simulink model "Task2_state_feedback_controller"  (R2023b)
settings: Solver=VariableStepAuto  StartTime=0.0  StopTime=0.02  RelTol=1e-3
values from neighbouring files (symbols this model uses):
  A = [-1.7  -0.25  0; 23  -30  20; 0  -250  -720]    [A.mat]
  B = [3  0; -103  0; 0  -790]    [B.mat]
  C = [0  1  0; 0  0  1]    [C.mat]
  K = K_bar*T    [Task1_pole_placement.m]    (also in Task2_LQR.m = R\B'*P; Task3_LQR_observer.m = R\B'*P; Task4_decoupling.m = F*[C(1,:)*(A+y11*eye(3));C(2,:)*(A+y21*eye(3))]; Task5_servo_control.m = R_ba\B_ba'*P)
settings Model: Creator=25039  LastModifiedBy=25039

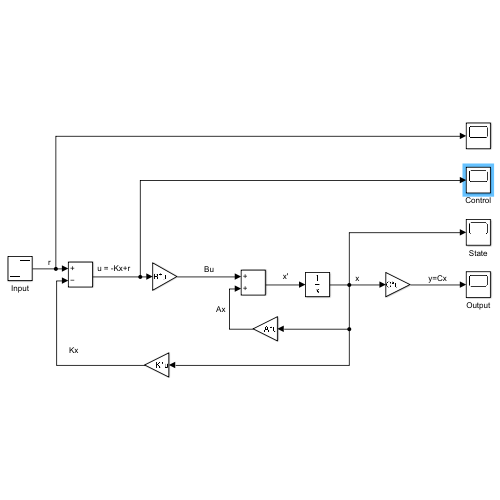
[thumbnail: Simulink's stored preview of the top-level diagram]
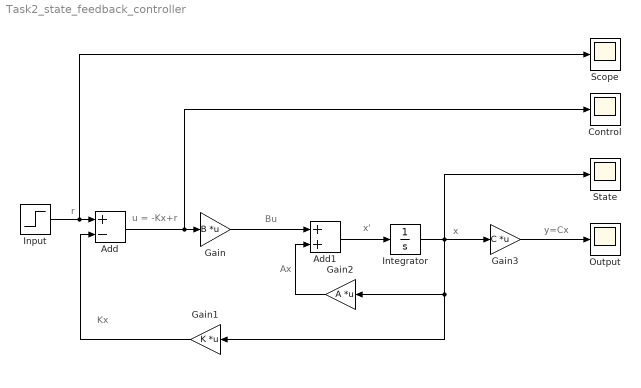
== system Task2_state_feedback_controller ==
  note: Kx
  note: y=Cx
  note: x
  note: x'
  note: Ax
  note: Bu
  note: u = -Kx+r
  note: r
  Add : Sum  Inputs=+-
  Add1 : Sum
  Control : Scope
  Gain : Gain  Gain=B  Multiplication=Matrix(K*u)
  Gain1 : Gain  Gain=K  Multiplication=Matrix(K*u)
  Gain2 : Gain  Gain=A  Multiplication=Matrix(K*u)
  Gain3 : Gain  Gain=C  Multiplication=Matrix(K*u)
  Input : Step  Time=0  Before=[0, 0]  After=[0, 0]
  Integrator : Integrator  InitialCondition=[1,100,200]
  Output : Scope
  Scope : Scope
  State : Scope
  wires:
  Input/1 -> Scope/1, Add/1
  Gain1/1 -> Add/2
  Add/1 -> Control/1, Gain/1
  Gain/1 -> Add1/1
  Gain2/1 -> Add1/2
  Add1/1 -> Integrator/1
  Integrator/1 -> State/1, Gain3/1, Gain1/1, Gain2/1
  Gain3/1 -> Output/1
